simulink model "quadtest"  (R2026a)
settings: Solver=FixedStepAuto  StopTime=inf  FixedStep=0.02  EnableMultiTasking=on
InitFcn:
  | init_tinympc_quad
values from neighbouring files (symbols this model uses):
  position = get_param(block,'Position')    [setup_tinympc_px4.m]
undefined symbols (not defined in the file or in its folder): acceleration, velocity, yaw, yawspeed
libraries: px4uORBlib x9
settings Model: ExtModeTrigDuration=10  Creator=Kristan  LastModifiedBy=imahajan
settings SolverCC: PositivePriorityOrder=on
settings OptimizationCC: InitFltsAndDblsToZero=on
settings HardwareCC: ProdLargestAtomicInteger=Long  ProdLargestAtomicFloat=Double  ProdHWDeviceType=ARM Compatible->ARM Cortex  TargetLongLongMode=on
settings SFSimCC: SimCustomHeaderCode=tinympc_interface.h  SimTargetLang=C++
settings SFSimCC: SimUserSources=|
  | wrapper/tinympc_interface.cpp
  | tinympc/TinyMPC/src/tinympc/admm.cpp
  | tinympc/TinyMPC/src/tinympc/tiny_api.cpp
  | tinympc/TinyMPC/src/tinympc/rho_benchmark.cpp
settings SFSimCC: SimUserIncludeDirs=|
  | ./wrapper
  | ./tinympc/TinyMPC/src
  | ./tinympc/TinyMPC/src/tinympc
  | ./tinympc/TinyMPC/include/Eigen
settings RTWCC: SystemTargetFile=ert.tlc  HardwareBoard=PX4 Host Target  TLCOptions="-aInlineSetEventsForThisBaseRateFcn=TLC_FALSE -aSuppressMultiTaskScheduler=TLC_FALSE  -aRateBasedStepFcn=0"  CustomHeaderCode=tinympc_interface.h  Toolchain=GNU Tools for PX4 Autopilots  PortableWordSizes=on  TargetLang=C++  Description=Embedded Coder
settings RTWCC: CustomInclude=|
  | ./wrapper
  | ./tinympc/TinyMPC/src
  | ./tinympc/TinyMPC/src/tinympc
  | ./tinympc/TinyMPC/include/Eigen
settings RTWCC: CustomSource=|
  | wrapper/tinympc_interface.cpp
  | tinympc/TinyMPC/src/tinympc/admm.cpp
  | tinympc/TinyMPC/src/tinympc/tiny_api.cpp
  | tinympc/TinyMPC/src/tinympc/rho_benchmark.cpp
settings ERTTargetCC: ExtModeTransport=2.0

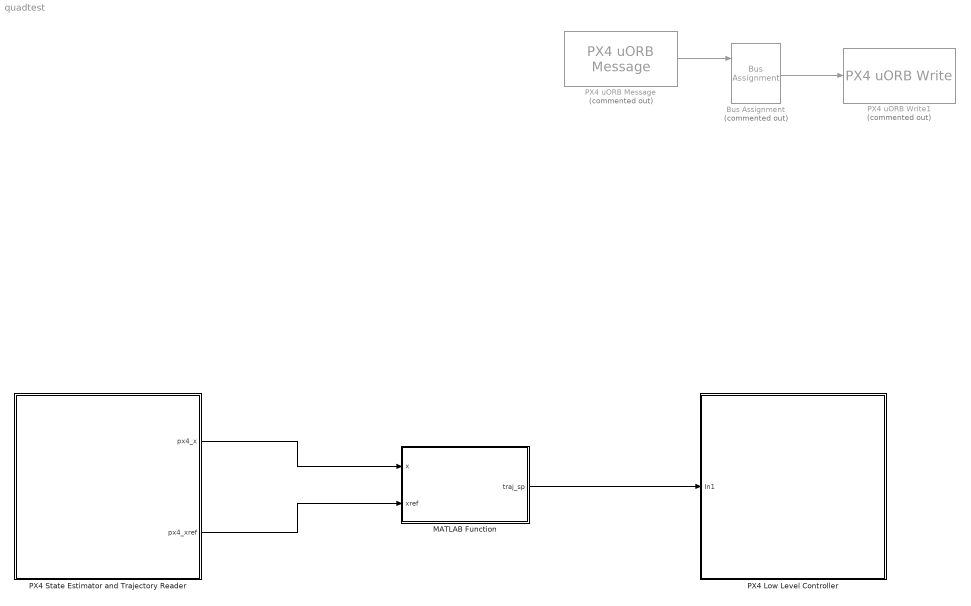
== system quadtest ==
  Bus Assignment : BusAssignment  Commented=on  AssignedSignals=xyz
  MATLAB Function : MATLAB Function  TreatAsAtomicUnit=on
  PX4 Low Level Controller : Subsystem
  "PX4 State Estimator and Trajectory Reader " : Subsystem
  PX4 uORB Message : px4uORBlib/PX4 uORB Message  Commented=on  uORBMsg=VehicleThrustSetpoint  uORBTopicName=vehicle_thrust_setpoint  isSingleTopicMsg=off  SampleTime=inf
  PX4 uORB Write1 : px4uORBlib/PX4 uORB Write  Commented=on  uORBMsg=VehicleThrustSetpoint  uORBTopicName=vehicle_thrust_setpoint  PublishOption=None  OutputPublishedInstanceNum=off  selectInstanceNum=1  OutputStatus=off  isSingleTopicMsg=off
  wires:
  PX4 uORB Message/1 -> Bus Assignment/1
  Bus Assignment/1 -> PX4 uORB Write1/1
  "PX4 State Estimator and Trajectory Reader "/1(px4_x) -> MATLAB Function/1(x)
  "PX4 State Estimator and Trajectory Reader "/2(px4_xref) -> MATLAB Function/2(xref)
  MATLAB Function/1(traj_sp) -> PX4 Low Level Controller/1(In1)

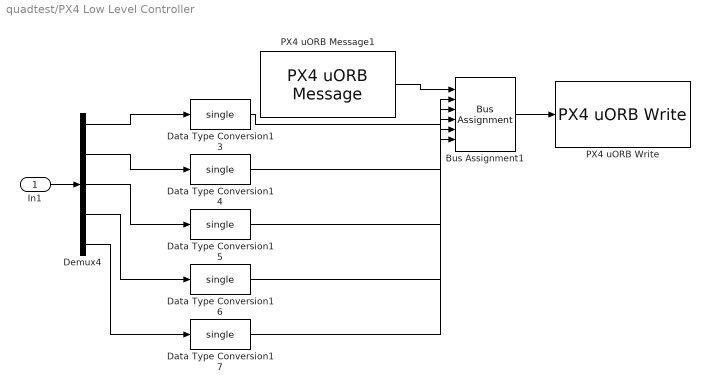
== system quadtest/PX4 Low Level Controller ==
  In1 : Inport
  Bus Assignment1 : BusAssignment  AssignedSignals=position,velocity,acceleration,yaw,yawspeed
  Data Type Conversion{13..17} (5 alike) : DataTypeConversion  OutDataTypeStr=single  SaturateOnIntegerOverflow=off  RndMeth=Floor
  Demux4 : Demux  Outputs=[3 3 3 1 1]
  PX4 uORB Message1 : px4uORBlib/PX4 uORB Message  uORBMsg=TrajectorySetpoint  uORBTopicName=trajectory_setpoint  isSingleTopicMsg=on  SampleTime=0.02
  PX4 uORB Write : px4uORBlib/PX4 uORB Write  uORBMsg=TrajectorySetpoint  uORBTopicName=trajectory_setpoint  PublishOption=None  OutputPublishedInstanceNum=off  selectInstanceNum=1  OutputStatus=off  isSingleTopicMsg=on
  wires:
  In1/1 -> Demux4/1
  PX4 uORB Message1/1 -> Bus Assignment1/1
  Demux4/1 -> Data Type Conversion13/1
  Data Type Conversion13/1 -> Bus Assignment1/2
  Demux4/2 -> Data Type Conversion14/1
  Data Type Conversion14/1 -> Bus Assignment1/3
  Demux4/3 -> Data Type Conversion15/1
  Data Type Conversion15/1 -> Bus Assignment1/4
  Demux4/4 -> Data Type Conversion16/1
  Data Type Conversion16/1 -> Bus Assignment1/5
  Demux4/5 -> Data Type Conversion17/1
  Data Type Conversion17/1 -> Bus Assignment1/6
  Bus Assignment1/1 -> PX4 uORB Write/1

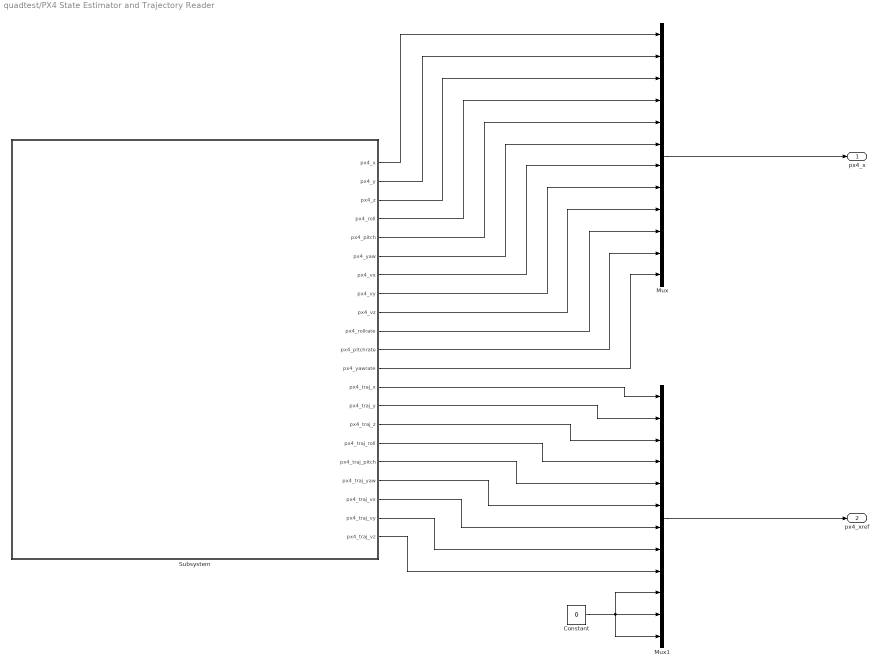
== system quadtest/PX4 State Estimator and Trajectory Reader  ==
  Constant : Constant  Value=0
  Mux : Mux  Inputs=12
  Mux1 : Mux  Inputs=12
  Subsystem : Subsystem
  px4_x : Outport
  px4_xref : Outport  Port=2
  wires:
  Subsystem/14(px4_traj_y) -> Mux1/2
  Subsystem/7(px4_vx) -> Mux/7
  Mux1/1 -> px4_xref/1
  Subsystem/13(px4_traj_x) -> Mux1/1
  Subsystem/8(px4_vy) -> Mux/8
  Subsystem/11(px4_pitchrate) -> Mux/11
  Subsystem/9(px4_vz) -> Mux/9
  Subsystem/5(px4_pitch) -> Mux/5
  Subsystem/10(px4_rollrate) -> Mux/10
  Subsystem/12(px4_yawrate) -> Mux/12
  Subsystem/15(px4_traj_z) -> Mux1/3
  Subsystem/16(px4_traj_roll) -> Mux1/4
  Mux/1 -> px4_x/1
  Subsystem/17(px4_traj_pitch) -> Mux1/5
  Subsystem/18(px4_traj_yaw) -> Mux1/6
  Subsystem/19(px4_traj_vx) -> Mux1/7
  Subsystem/20(px4_traj_vy) -> Mux1/8
  Subsystem/21(px4_traj_vz) -> Mux1/9
  Subsystem/1(px4_x) -> Mux/1
  Subsystem/2(px4_y) -> Mux/2
  Subsystem/4(px4_roll) -> Mux/4
  Subsystem/3(px4_z) -> Mux/3
  Constant/1 -> Mux1/12, Mux1/11, Mux1/10
  Subsystem/6(px4_yaw) -> Mux/6

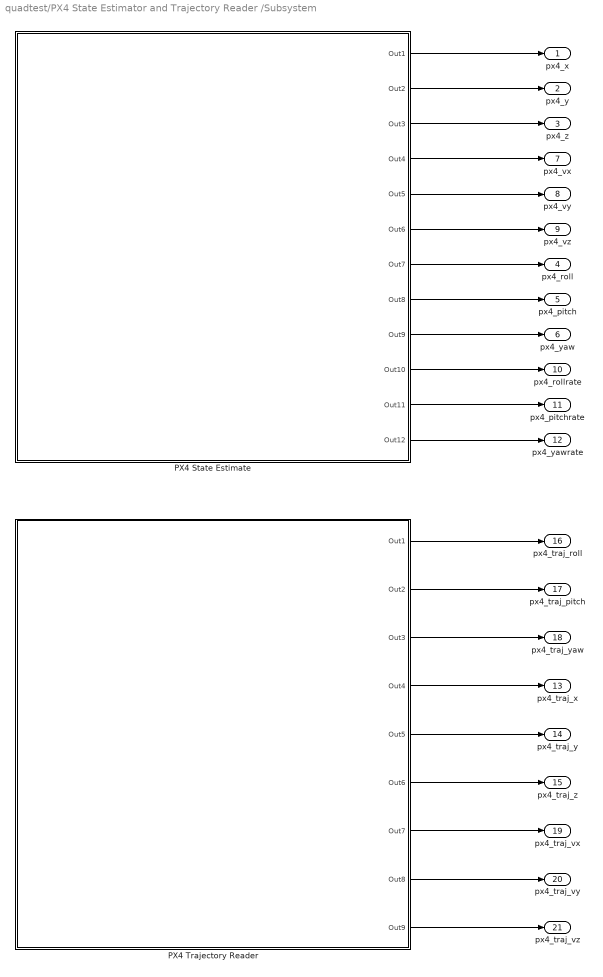
== system quadtest/PX4 State Estimator and Trajectory Reader /Subsystem ==
  PX4 State Estimate : Subsystem
  PX4 Trajectory Reader : Subsystem
  px4_x : Outport
  px4_y : Outport  Port=2
  px4_z : Outport  Port=3
  px4_roll : Outport  Port=4
  px4_pitch : Outport  Port=5
  px4_yaw : Outport  Port=6
  px4_vx : Outport  Port=7
  px4_vy : Outport  Port=8
  px4_vz : Outport  Port=9
  px4_rollrate : Outport  Port=10
  px4_pitchrate : Outport  Port=11
  px4_yawrate : Outport  Port=12
  px4_traj_x : Outport  Port=13
  px4_traj_y : Outport  Port=14
  px4_traj_z : Outport  Port=15
  px4_traj_roll : Outport  Port=16
  px4_traj_pitch : Outport  Port=17
  px4_traj_yaw : Outport  Port=18
  px4_traj_vx : Outport  Port=19
  px4_traj_vy : Outport  Port=20
  px4_traj_vz : Outport  Port=21
  wires:
  PX4 Trajectory Reader/1(Out1) -> px4_traj_roll/1
  PX4 Trajectory Reader/2(Out2) -> px4_traj_pitch/1
  PX4 Trajectory Reader/3(Out3) -> px4_traj_yaw/1
  PX4 Trajectory Reader/4(Out4) -> px4_traj_x/1
  PX4 Trajectory Reader/5(Out5) -> px4_traj_y/1
  PX4 Trajectory Reader/6(Out6) -> px4_traj_z/1
  PX4 Trajectory Reader/7(Out7) -> px4_traj_vx/1
  PX4 Trajectory Reader/8(Out8) -> px4_traj_vy/1
  PX4 Trajectory Reader/9(Out9) -> px4_traj_vz/1
  PX4 State Estimate/1(Out1) -> px4_x/1
  PX4 State Estimate/2(Out2) -> px4_y/1
  PX4 State Estimate/3(Out3) -> px4_z/1
  PX4 State Estimate/4(Out4) -> px4_vx/1
  PX4 State Estimate/5(Out5) -> px4_vy/1
  PX4 State Estimate/6(Out6) -> px4_vz/1
  PX4 State Estimate/7(Out7) -> px4_roll/1
  PX4 State Estimate/8(Out8) -> px4_pitch/1
  PX4 State Estimate/9(Out9) -> px4_yaw/1
  PX4 State Estimate/10(Out10) -> px4_rollrate/1
  PX4 State Estimate/11(Out11) -> px4_pitchrate/1
  PX4 State Estimate/12(Out12) -> px4_yawrate/1

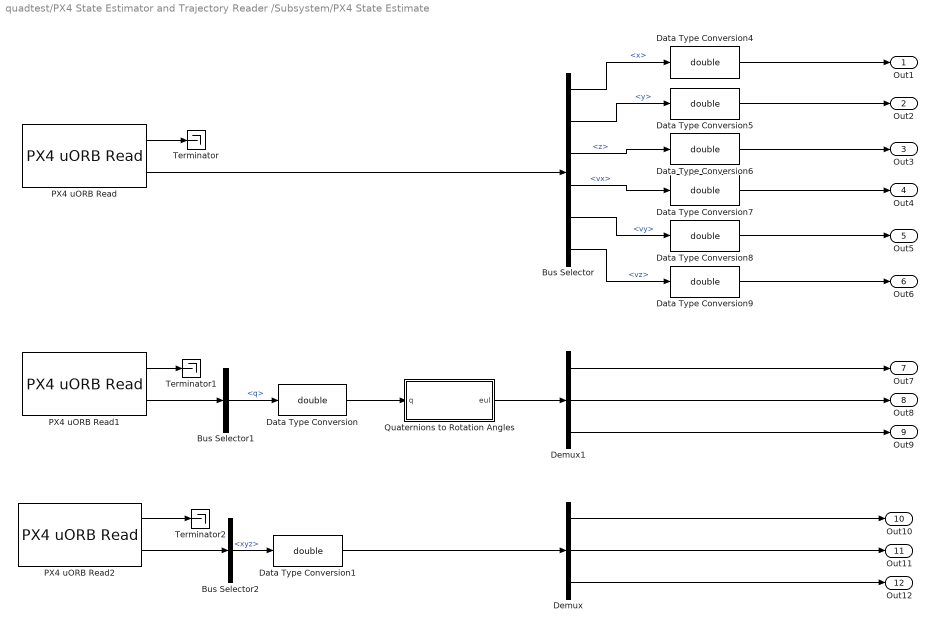
== system quadtest/PX4 State Estimator and Trajectory Reader /Subsystem/PX4 State Estimate ==
  Bus Selector : BusSelector  OutputSignals=x,y,z,vx,vy,vz
  Bus Selector1 : BusSelector  OutputSignals=q
  Bus Selector2 : BusSelector  OutputSignals=xyz
  Data Type Conversion{,1,4..9} (8 alike) : DataTypeConversion  OutDataTypeStr=double  SaturateOnIntegerOverflow=off  RndMeth=Floor
  Demux : Demux  Outputs=3
  Demux1 : Demux  Outputs=3
  PX4 uORB Read : px4uORBlib/PX4 uORB Read  uORBMsg=VehicleLocalPosition  uORBTopicName=vehicle_local_position  SubscribeNonZeroInstance=off  selectInstanceNum=1  SampleTime=0.02  isSingleTopicMsg=off  BlockingMode=off  BlockTimeout=1e-3
  PX4 uORB Read1 : px4uORBlib/PX4 uORB Read  uORBMsg=VehicleAttitude  uORBTopicName=vehicle_attitude  SubscribeNonZeroInstance=off  selectInstanceNum=1  SampleTime=0.02  isSingleTopicMsg=off  BlockingMode=off  BlockTimeout=1e-3
  PX4 uORB Read2 : px4uORBlib/PX4 uORB Read  uORBMsg=VehicleAngularVelocity  uORBTopicName=vehicle_angular_velocity  SubscribeNonZeroInstance=off  selectInstanceNum=1  SampleTime=0.02  isSingleTopicMsg=off  BlockingMode=off  BlockTimeout=1e-3
  Quaternions to Rotation Angles : MATLAB Function  TreatAsAtomicUnit=on
  Terminator : Terminator
  Terminator1 : Terminator
  Terminator2 : Terminator
  Out1 : Outport
  Out2 : Outport  Port=2
  Out3 : Outport  Port=3
  Out4 : Outport  Port=4
  Out5 : Outport  Port=5
  Out6 : Outport  Port=6
  Out7 : Outport  Port=7
  Out8 : Outport  Port=8
  Out9 : Outport  Port=9
  Out10 : Outport  Port=10
  Out11 : Outport  Port=11
  Out12 : Outport  Port=12
  wires:
  Data Type Conversion9/1 -> Out6/1
  Data Type Conversion8/1 -> Out5/1
  Bus Selector2/1 -> Data Type Conversion1/1  "<xyz>"
  Bus Selector1/1 -> Data Type Conversion/1  "<q>"
  Data Type Conversion6/1 -> Out3/1
  PX4 uORB Read2/2 -> Bus Selector2/1
  PX4 uORB Read1/1 -> Terminator1/1
  Bus Selector/3 -> Data Type Conversion6/1  "<z>"
  PX4 uORB Read2/1 -> Terminator2/1
  Bus Selector/6 -> Data Type Conversion9/1  "<vz>"
  Bus Selector/5 -> Data Type Conversion8/1  "<vy>"
  PX4 uORB Read1/2 -> Bus Selector1/1
  Bus Selector/1 -> Data Type Conversion4/1  "<x>"
  PX4 uORB Read/1 -> Terminator/1
  PX4 uORB Read/2 -> Bus Selector/1
  Data Type Conversion1/1 -> Demux/1
  Demux1/1 -> Out7/1
  Bus Selector/4 -> Data Type Conversion7/1  "<vx>"
  Bus Selector/2 -> Data Type Conversion5/1  "<y>"
  Demux1/2 -> Out8/1
  Data Type Conversion4/1 -> Out1/1
  Data Type Conversion5/1 -> Out2/1
  Demux1/3 -> Out9/1
  Data Type Conversion7/1 -> Out4/1
  Demux/1 -> Out10/1
  Demux/2 -> Out11/1
  Demux/3 -> Out12/1
  Data Type Conversion/1 -> Quaternions to Rotation Angles/1(q)
  Quaternions to Rotation Angles/1(eul) -> Demux1/1

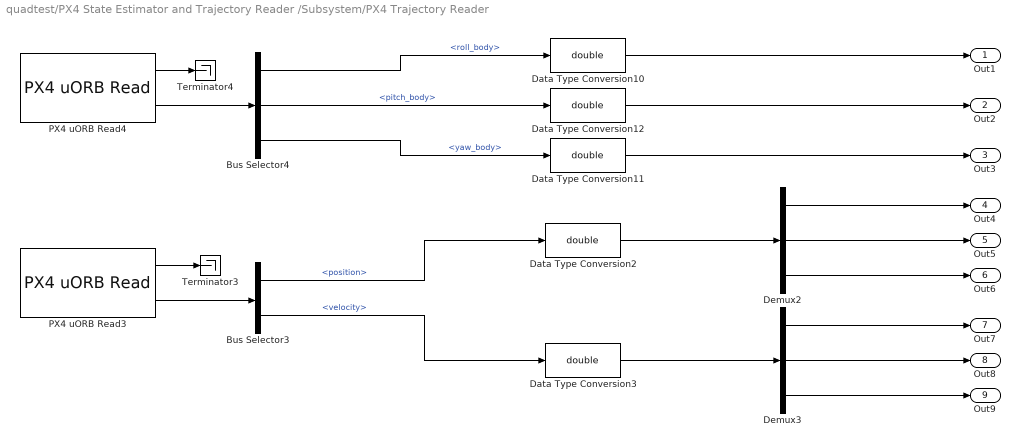
== system quadtest/PX4 State Estimator and Trajectory Reader /Subsystem/PX4 Trajectory Reader ==
  Bus Selector3 : BusSelector  OutputSignals=position,velocity
  Bus Selector4 : BusSelector  OutputSignals=roll_body,pitch_body,yaw_body
  Data Type Conversion{2..3,10..12} (5 alike) : DataTypeConversion  OutDataTypeStr=double  SaturateOnIntegerOverflow=off  RndMeth=Floor
  Demux2 : Demux  Outputs=3
  Demux3 : Demux  Outputs=3
  PX4 uORB Read3 : px4uORBlib/PX4 uORB Read  uORBMsg=TrajectorySetpoint  uORBTopicName=TrajectorySetpoint  SubscribeNonZeroInstance=off  selectInstanceNum=1  SampleTime=0.02  isSingleTopicMsg=off  BlockingMode=off  BlockTimeout=1e-3
  PX4 uORB Read4 : px4uORBlib/PX4 uORB Read  uORBMsg=VehicleAttitudeSetpoint  uORBTopicName=vehicle_attitude_setpoint  SubscribeNonZeroInstance=off  selectInstanceNum=1  SampleTime=0.02  isSingleTopicMsg=off  BlockingMode=off  BlockTimeout=1e-3
  Terminator3 : Terminator
  Terminator4 : Terminator
  Out1 : Outport
  Out2 : Outport  Port=2
  Out3 : Outport  Port=3
  Out4 : Outport  Port=4
  Out5 : Outport  Port=5
  Out6 : Outport  Port=6
  Out7 : Outport  Port=7
  Out8 : Outport  Port=8
  Out9 : Outport  Port=9
  wires:
  Data Type Conversion3/1 -> Demux3/1
  Demux3/2 -> Out8/1
  Bus Selector3/2 -> Data Type Conversion3/1  "<velocity>"
  Demux3/3 -> Out9/1
  Bus Selector4/2 -> Data Type Conversion12/1  "<pitch_body>"
  PX4 uORB Read4/2 -> Bus Selector4/1
  PX4 uORB Read3/2 -> Bus Selector3/1
  Data Type Conversion2/1 -> Demux2/1
  Bus Selector4/1 -> Data Type Conversion10/1  "<roll_body>"
  PX4 uORB Read3/1 -> Terminator3/1
  PX4 uORB Read4/1 -> Terminator4/1
  Bus Selector3/1 -> Data Type Conversion2/1  "<position>"
  Bus Selector4/3 -> Data Type Conversion11/1  "<yaw_body>"
  Data Type Conversion10/1 -> Out1/1
  Demux2/2 -> Out5/1
  Demux2/3 -> Out6/1
  Demux2/1 -> Out4/1
  Demux3/1 -> Out7/1
  Data Type Conversion11/1 -> Out3/1
  Data Type Conversion12/1 -> Out2/1

== matlab function quadtest/MATLAB Function ==
  data: x input size=[1 12]; traj_sp output size=[1 11]; xref input size=[12 1]
function traj_sp = TinyMPC_Controller(x, xref)
%#codegen
% TinyMPC hover outer loop (guidance MPC).
%
% x is [x y z roll pitch yaw vx vy vz p q r] in PX4 NED/local frame.
% The hover reference is latched 1 m above the state at the first
% step after the app engages, so it is immune to the EKF z-origin
% drift that accumulates while grounded.
%
% MPC_Step_Plan returns u0 = [ax ay az yawspeed] plus the one-step-
% ahead predicted state x1. We publish the MPC PLAN (x1 position and
% velocity, u0 acceleration feed-forward, x1 yaw, u0 yawspeed) as
% [position(1x3), velocity(1x3), acceleration(1x3), yaw, yawspeed],
% so PX4's position controller tracks TinyMPC's trajectory while
% keeping acceleration-to-attitude conversion, attitude control,
% rate control, and the mixer downstream.

persistent ref_pos ref_yaw have_ref last_traj
if isempty(have_ref)
    have_ref = false;
    ref_pos = zeros(3,1,'single');
    ref_yaw = single(0.0);
    last_traj = zeros(1,11,'single');
end

mpc_u = zeros(4,1,'single');
x_next = zeros(12,1,'single');
x_single = single(x);
xref_in = single(xref);

if ~have_ref && all(isfinite(x_single(1:3)))
    ref_pos = [x_single(1); x_single(2); x_single(3) - single(1.0)];
    ref_yaw = x_single(6);
    last_traj = [x_single(1), x_single(2), x_single(3), ...
                 single(0.0), single(0.0), single(0.0), ...
                 single(0.0), single(0.0), single(0.0), ...
                 ref_yaw, single(0.0)];
    have_ref = true;
end

hover_ref = zeros(12,1,'single');
hover_ref(1:3) = ref_pos;
hover_ref(6) = ref_yaw;

% Keep xref connected for code-generation shape inference and future
% external trajectory mode, but force this first demo to a 1 m hover.
if false
    hover_ref = xref_in;
end

coder.cinclude('tinympc_interface.h');

coder.ceval('MPC_Step_Plan', ...
            coder.rref(x_single), ...
            coder.rref(hover_ref), ...
            coder.wref(mpc_u), ...
            coder.wref(x_next));

traj_single = zeros(1,11,'single');
traj_single(1) = x_next(1);
traj_single(2) = x_next(2);
traj_single(3) = x_next(3);
traj_single(4) = x_next(7);
traj_single(5) = x_next(8);
traj_single(6) = x_next(9);
traj_single(7) = min(max(mpc_u(1), single(-4.0)), single(4.0));
traj_single(8) = min(max(mpc_u(2), single(-4.0)), single(4.0));
traj_single(9) = min(max(mpc_u(3), single(-4.0)), single(4.0));
traj_single(10) = x_next(6);
traj_single(11) = min(max(mpc_u(4), single(-1.0)), single(1.0));

% Solver-failure guard: never publish non-finite setpoints; hold the
% last good plan instead (PX4 then tracks the last planned point).
if all(isfinite(traj_single))
    last_traj = traj_single;
else
    traj_single = last_traj;
end

traj_sp = double(traj_single);

end

== matlab function quadtest/PX4 State Estimator and Trajectory Reader /Subsystem/PX4 State Estimate/Quaternions to Rotation Angles ==
  data: q input; eul output
function eul = fcn(q)
%#codegen
% q is PX4 vehicle_attitude.q ordered as [w x y z].
qw = q(1);
qx = q(2);
qy = q(3);
qz = q(4);

sinr_cosp = 2.0 * (qw*qx + qy*qz);
cosr_cosp = 1.0 - 2.0 * (qx*qx + qy*qy);
roll = atan2(sinr_cosp, cosr_cosp);

sinp = 2.0 * (qw*qy - qz*qx);
if sinp >= 1.0
    pitch = pi / 2.0;
elseif sinp <= -1.0
    pitch = -pi / 2.0;
else
    pitch = asin(sinp);
end

siny_cosp = 2.0 * (qw*qz + qx*qy);
cosy_cosp = 1.0 - 2.0 * (qy*qy + qz*qz);
yaw = atan2(siny_cosp, cosy_cosp);

eul = [roll; pitch; yaw];
